simulink model "torque_robot"  (R2025b)
settings: Solver=VariableStepAuto  StartTime=0.0  StopTime=10.0  MaxStep=0.2  RelTol=1e-3
PostLoadFcn:
  | rigid_body = importrobot('urdf\lbr_description\urdf\iiwa7.urdf');
  | rigid_body.DataFormat = 'column';
  | rigid_body.Gravity = [0 0 -9.81];
  | init_joint_pos = [0 75 0 -94 0 -81 0] / 180 * pi;
  | robot = get_robot_chain(rigid_body);
  | n = robot.dof;
  | T_init = forward_kin_general(robot, init_joint_pos);
  | T_end = T_init;
  | T_end(3,4) = T_end(3,4) + 0.5;
  | Fext = zeros(6,7);
libraries: my_library x3, robotcorelib x2
settings Model: Creator=Junch  LastModifiedBy=Junch

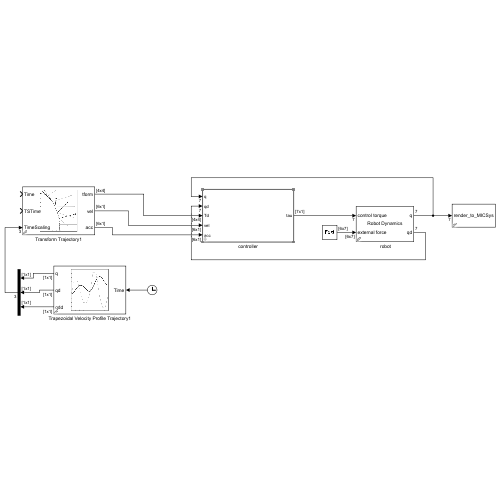
[thumbnail: Simulink's stored preview of the top-level diagram]
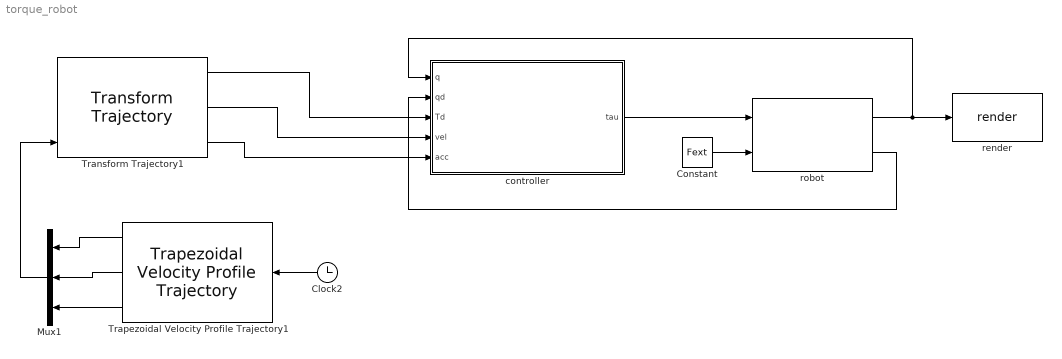
== system torque_robot ==
  " robot" : my_library/   robot=robot  init_pos=init_joint_pos  init_vel=zeros(1,robot.dof)
      settings: SourceProductName=MyLibrary
  Clock2 : Clock
  Constant : Constant  Value=Fext
  Mux1 : Mux  Inputs=3
  Transform Trajectory1 : robotcorelib/Transform Trajectory  WaypointSource=Internal  T0=T_init  TF=T_end  TimeInterval=[0, 1]  CustomTimeScaling=on  ParameterSource=External  TSTime=2:0.1:3  TimeScaling=[ 0:0.1:1; ones( 1, 11 ); zeros( 1, 11 ) ]  SimulateUsing=Interpreted execution
      settings: LibrarySourceBlock=robotutilslib/Transform Trajectory
  Trapezoidal Velocity Profile Trajectory1 : robotcorelib/Trapezoidal Velocity Profile Trajectory  WaypointSource=Internal  Waypoints=[ 0, 1]  NumParams=1  Parameter1=End Time  Parameter2=End Time  ParameterSource=Internal  PeakVelocity=[ 2; 2 ]  Acceleration=[ 1; 2 ]  EndTime=10  AccelTime=[ 1; 2 ]  SimulateUsing=Interpreted execution
  controller : Subsystem  mask{robot=robot, Bx=100*ones(1, 6), Kx=1500*ones(1, 6), Ki=0*ones(1,6), Bn=2*ones(1,robot.dof), Kn=2*ones(1,robot.dof), method=PD+, Y=1*ones(1,robot.dof)}
      mask prompts: Y "观测器增益"
      mask init:
      | switch method
      |     case 'PD'
      |         mode = int32(1);
      | 
      |     case 'PD+'
      |         mode = int32(2);
      | 
      |     otherwise
      |         mode = int32(3);
      | end
      mask TypeOptions method: PD | PD+ | Passivity
      mask DialogControl ParameterGroupVar Prompt: 参数
  render : my_library/render  Ts=0.05
      settings: SourceProductName=MyLibrary
  wires:
  " robot"/1 -> controller/1(q), render/1
  " robot"/2 -> controller/2(qd)
  controller/1(tau) -> " robot"/1
  Clock2/1 -> Trapezoidal Velocity Profile Trajectory1/1
  Trapezoidal Velocity Profile Trajectory1/3 -> Mux1/3
  Mux1/1 -> Transform Trajectory1/3
  Trapezoidal Velocity Profile Trajectory1/1 -> Mux1/1
  Transform Trajectory1/1 -> controller/3(Td)
  Transform Trajectory1/3 -> controller/5(acc)
  Transform Trajectory1/2 -> controller/4(vel)
  Trapezoidal Velocity Profile Trajectory1/2 -> Mux1/2
  Constant/1 -> " robot"/2

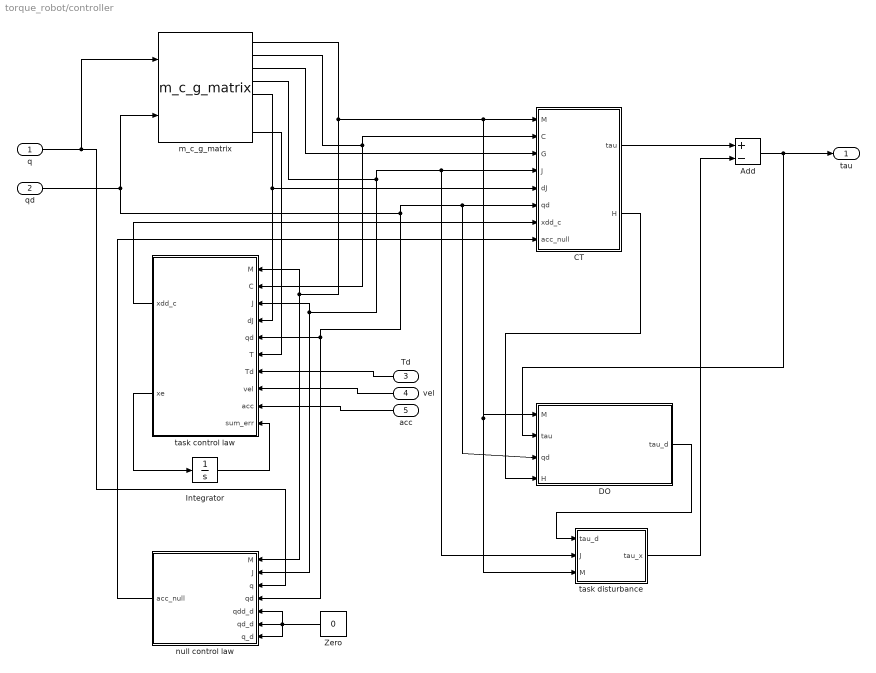
== system torque_robot/controller ==
  q : Inport
  qd : Inport  Port=2
  Td : Inport  Port=3
  vel : Inport  Port=4
  acc : Inport  Port=5
  Add : Sum  Inputs=+-
  CT : MATLAB Function  TreatAsAtomicUnit=on
  DO : Subsystem  mask{Y=Y}
      mask prompts: Y "观测器增益"
      mask DialogControl ParameterGroupVar Prompt: 参数
  Integrator : Integrator
  Zero : Constant  Value=0  OutDataTypeStr=Inherit: Inherit via back propagation
  m_c_g_matrix : my_library/m_c_g_matrix  robot=robot
  null control law : MATLAB Function  TreatAsAtomicUnit=on  mask{Bn=Bn, Kn=Kn}
  task control law : MATLAB Function  TreatAsAtomicUnit=on  mask{Bx=Bx, Kx=Kx, Ki=Ki, mode=mode}
  "task disturbance " : MATLAB Function  TreatAsAtomicUnit=on
  tau : Outport
  wires:
  m_c_g_matrix/2 -> task control law/2(C), CT/2(C)
  m_c_g_matrix/5 -> task control law/4(dJ), CT/5(dJ)
  null control law/1(acc_null) -> CT/8(acc_null)
  m_c_g_matrix/1 -> null control law/1(M), task control law/1(M), "task disturbance "/3(M), DO/1(M), CT/1(M)
  qd/1 -> null control law/4(qd), task control law/5(qd), DO/3(qd), CT/6(qd), m_c_g_matrix/2
  Td/1 -> task control law/7(Td)
  vel/1 -> task control law/8(vel)
  m_c_g_matrix/3 -> CT/3(G)
  m_c_g_matrix/4 -> null control law/2(J), task control law/3(J), "task disturbance "/2(J), CT/4(J)
  m_c_g_matrix/8 -> task control law/6(T)
  acc/1 -> task control law/9(acc)
  q/1 -> null control law/3(q), m_c_g_matrix/1
  Zero/1 -> null control law/7(q_d), null control law/6(qd_d), null control law/5(qdd_d)
  task control law/1(xdd_c) -> CT/7(xdd_c)
  task control law/2(xe) -> Integrator/1
  Integrator/1 -> task control law/10(sum_err)
  CT/2(H) -> DO/4(H)
  CT/1(tau) -> Add/1
  Add/1 -> tau/1, DO/2(tau)
  DO/1(tau_d) -> "task disturbance "/1(tau_d)
  "task disturbance "/1(tau_x) -> Add/2

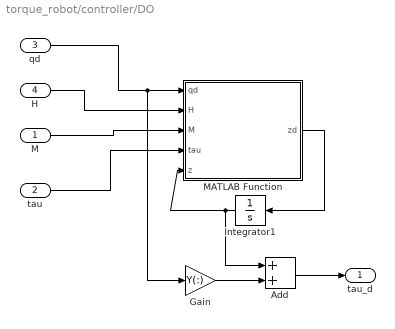
== system torque_robot/controller/DO ==
  M : Inport
  tau : Inport  Port=2
  qd : Inport  Port=3
  H : Inport  Port=4
  Add : Sum
  Gain : Gain  Gain=Y(:)
  Integrator1 : Integrator
  MATLAB Function : MATLAB Function  TreatAsAtomicUnit=on
  tau_d : Outport
  wires:
  qd/1 -> Gain/1, MATLAB Function/1(qd)
  MATLAB Function/1(zd) -> Integrator1/1
  Integrator1/1 -> MATLAB Function/5(z), Add/1
  H/1 -> MATLAB Function/2(H)
  M/1 -> MATLAB Function/3(M)
  tau/1 -> MATLAB Function/4(tau)
  Gain/1 -> Add/2
  Add/1 -> tau_d/1

== matlab function torque_robot/controller/CT ==
  data: M input; C input; G input; J input; dJ input; qd input; xdd_c input; acc_null input; tau output; H output
function [tau, H] = fcn(M, C, G, J, dJ, qd,xdd_c, acc_null)
%#codegen
acc_task = pinv_J_x(J, M, xdd_c - dJ * qd);
qdd_c = acc_task + acc_null;
H =  C * qd + G;
tau = M * qdd_c + H;

== matlab function torque_robot/controller/task control law ==
  data: M input; C input; J input; dJ input; qd input; T input; Td input; xdd_c output; vel input; acc input; sum_err input; Bx parameter; Kx parameter; xe output; Ki parameter; mode parameter
function [xdd_c, xe] = fcn(M, C, J, dJ, qd,  T, Td, vel, acc, sum_err, Bx, Kx, Ki, mode)
R = T(1:3,1:3);
Rd = Td(1:3,1:3);
p = T(1:3, 4);
pd = Td(1:3, 4);
V = J * qd;
xe = [logR(R' * Rd)'; R' * (pd - p)];
xed = [R' * vel(1:3); R' * vel(4:6)] - V;
xdd_d = [R' * (acc(1:3) - cross(R * V(1:3), vel(1:3))); R' * (acc(4:6) - cross(R * V(1:3), vel(4:6)))];
if mode == 1
%% PD
xdd_c = xdd_d + Kx(:) .* xe + Bx(:) .* xed;
elseif mode == 2
%% PD+
xdd_c = xdd_d + A_x_inv(J, M) * ((Mu_x(J, M, dJ, C) + diag(Bx)) * xed + Kx(:) .* xe + Ki(:) .* sum_err);
else
%% Passivity
s = xed + Kx(:) .* xe;
sum_s_err = xe + Kx(:) .* sum_err;
xdd_c = xdd_d + Kx(:) .* xed + A_x_inv(J, M) * ((Mu_x(J, M, dJ, C) + Bx(:))) * s + Ki(:) .* sum_s_err;
end

== matlab function torque_robot/controller/null control law ==
  data: M input; J input; q input; qd input; qdd_d input; acc_null output; qd_d input; q_d input; Bn parameter; Kn parameter
function acc_null = fcn(M, J, q, qd, qdd_d, qd_d, q_d, Bn, Kn)
%#codegen
qed = qd_d - qd;
qe = q_d - q;
acc_null = null_proj(J, M, qdd_d + M \ (Bn(:) .* qed + Kn(:) .* qe));

== matlab function torque_robot/controller/task disturbance  ==
  data: tau_d input; tau_x output; J input; M input
function tau_x = fcn(tau_d, J, M)

tau_x = J' * ((J * (M \ J')) \ J) * (M \ tau_d) ;

== matlab function torque_robot/controller/DO/MATLAB Function ==
  data: qd input; zd output; H input; M input; tau input; z input; Y parameter
function zd = fcn(qd, H, M, tau, z, Y)
%#codegen
p = Y(:) .* qd;
zd = Y(:) .* (M \ (H - tau - z - p));
